simulink model "Simulation"  (R2024b)
settings: Solver=ode45  StartTime=0.0  StopTime=10.0  RelTol=1e-6
values from neighbouring files (symbols this model uses):
  B0 = 0.0001    [Constants.m]
  J = 0.001    [Constants.m]
  Kb = 0.05    [Constants.m]
  KT = 0.015    [Constants.m]
  La = 0.5    [Constants.m]
  Ra = 2.0    (= 2)    [Constants.m]
settings Model: Creator=makar  LastModifiedBy=makar

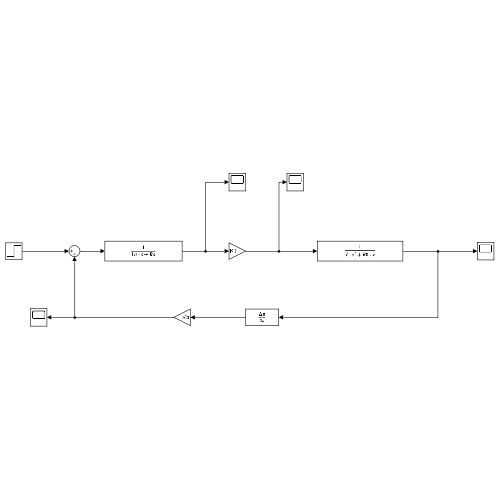
[thumbnail: Simulink's stored preview of the top-level diagram]
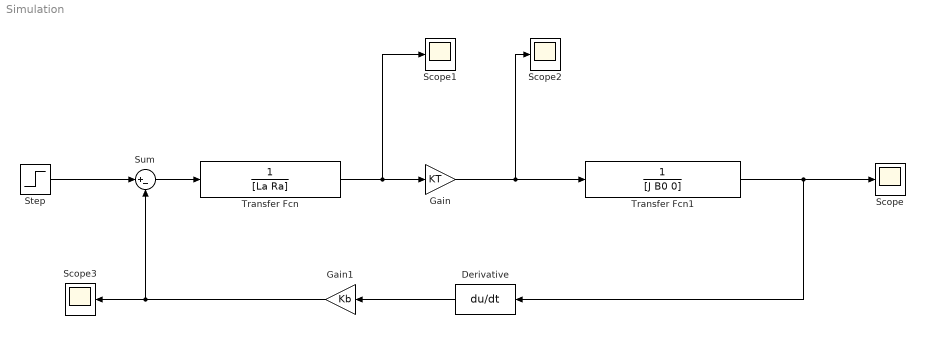
== system Simulation ==
  Derivative : Derivative
  Gain : Gain  Gain=KT
  Gain1 : Gain  Gain=Kb
  Scope{,1..3} (4 alike) : Scope
  Step : Step  Time=0  After=5  SampleTime=0
  Sum : Sum  Inputs=|+-
  Transfer Fcn : TransferFcn  Denominator=[La Ra]
  Transfer Fcn1 : TransferFcn  Denominator=[J B0 0]
  wires:
  Step/1 -> Sum/1
  Sum/1 -> Transfer Fcn/1
  Transfer Fcn/1 -> Gain/1, Scope1/1
  Gain/1 -> Scope2/1, Transfer Fcn1/1
  Transfer Fcn1/1 -> Derivative/1, Scope/1
  Gain1/1 -> Scope3/1, Sum/2
  Derivative/1 -> Gain1/1
